simulink model "histogram_AXIS_TMI_2pix"  (R2015b)
settings: Solver=FixedStepDiscrete  SolverMode=SingleTasking  StartTime=0.0  StopTime=StartTime  FixedStep=1  RelTol=1e-3
values from neighbouring files (symbols this model uses):
  Nb_bin = 128    [Histogram_aldec_validation.m]    (also in Histogram_init.m = 1024; Histogram_init_20163.m; Histogram_init_validation.m)
  Ts = 1    [Histogram_aldec_validation.m]    (also in Histogram_init.m; Histogram_init_20163.m; Histogram_init_validation.m)
libraries: xbsIndex_r4 x128
settings Model: Creator=jboulet  LastModifiedBy=laboutilis
settings DataIOCC: SaveFormat=Array  SignalLoggingSaveFormat=ModelDataLogs
settings OptimizationCC: ExpressionDepthLimit=2147483647  InitFltsAndDblsToZero=on
settings DebuggingCC: AlgebraicLoopMsg=none  UnderspecifiedInitializationDetection=Classic  MergeDetectMultiDrivingBlocksExec=none  FcnCallInpInsideContextMsg=UseLocalSettings  UnconnectedInputMsg=none  UnconnectedOutputMsg=none  UnconnectedLineMsg=none  StateNameClashWarn=warning
settings HardwareCC: ProdBitPerPointer=32  ProdLargestAtomicFloat=None  ProdIntDivRoundTo=Undefined  ProdEndianess=Unspecified  ProdWordSize=32  ProdHWDeviceType=32-bit Generic
settings GRTTargetCC: GeneratePreprocessorConditionals=Disable all  CombineOutputUpdateFcns=off  GRTInterface=on
settings ConfigComp: CovModelRefEnable=Off

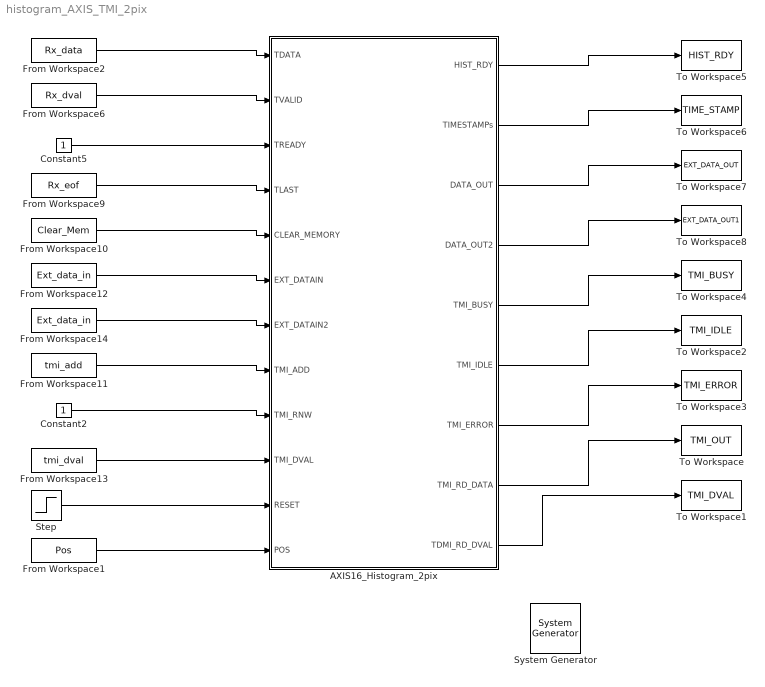
== system histogram_AXIS_TMI_2pix ==
  " System Generator" : xbsIndex_r4/ System Generator  Tag=genX  xilinxfamily=kintex7  part=xc7k160t  speed=-1  package=fbg676  synthesis_tool=Vivado  clock_wrapper=Clock Enables  directory=D:/Telops/FIR-00251-Proc/src/AEC/HDL/2pix_netlist_160  proj_type=Vivado  Synth_file=Vivado Synthesis Defaults  Impl_file=Vivado Implementation Defaults  testbench=off  simulink_period=1  sysclk_period=6.25  dcm_input_clock_period=10  incr_netlist=off  trim_vbits=Everywhere in SubSystem  dbl_ovrd=According to Block Masks  core_generation=According to Block Masks  run_coregen=off  deprecated_control=off  eval_field=0  block_type=sysgen
  AXIS16_Histogram_2pix : Subsystem
  Constant2 : Constant
  Constant5 : Constant
  From Workspace1 : FromWorkspace  VariableName=Pos  SampleTime=Ts  Interpolate=off  OutputAfterFinalValue=Holding final value
  From Workspace10 : FromWorkspace  VariableName=Clear_Mem  SampleTime=Ts  Interpolate=off  OutputAfterFinalValue=Setting to zero
  From Workspace11 : FromWorkspace  VariableName=tmi_add  SampleTime=Ts  Interpolate=off  OutputAfterFinalValue=Holding final value
  From Workspace12 : FromWorkspace  VariableName=Ext_data_in  SampleTime=Ts  Interpolate=off  OutputAfterFinalValue=Setting to zero
  From Workspace13 : FromWorkspace  VariableName=tmi_dval  SampleTime=Ts  Interpolate=off  OutputAfterFinalValue=Holding final value
  From Workspace14 : FromWorkspace  VariableName=Ext_data_in  SampleTime=Ts  Interpolate=off  OutputAfterFinalValue=Setting to zero
  From Workspace2 : FromWorkspace  VariableName=Rx_data  SampleTime=Ts  Interpolate=off  OutputAfterFinalValue=Setting to zero
  From Workspace6 : FromWorkspace  VariableName=Rx_dval  SampleTime=Ts  Interpolate=off  OutputAfterFinalValue=Setting to zero
  From Workspace9 : FromWorkspace  VariableName=Rx_eof  SampleTime=Ts  Interpolate=off  OutputAfterFinalValue=Setting to zero
  Step : Step  Time=5  Before=1  After=0  SampleTime=Ts
  To Workspace : ToWorkspace  VariableName=TMI_OUT  SampleTime=-1
  To Workspace1 : ToWorkspace  VariableName=TMI_DVAL  SampleTime=-1
  To Workspace2 : ToWorkspace  VariableName=TMI_IDLE  SampleTime=-1
  To Workspace3 : ToWorkspace  VariableName=TMI_ERROR  SampleTime=-1
  To Workspace4 : ToWorkspace  VariableName=TMI_BUSY  SampleTime=-1
  To Workspace5 : ToWorkspace  VariableName=HIST_RDY  SampleTime=-1
  To Workspace6 : ToWorkspace  VariableName=TIME_STAMP  SampleTime=-1
  To Workspace7 : ToWorkspace  VariableName=EXT_DATA_OUT  SampleTime=-1
  To Workspace8 : ToWorkspace  VariableName=EXT_DATA_OUT1  SampleTime=-1
  wires:
  From Workspace2/1 -> AXIS16_Histogram_2pix/1(TDATA)
  From Workspace6/1 -> AXIS16_Histogram_2pix/2(TVALID)
  Constant5/1 -> AXIS16_Histogram_2pix/3(TREADY)
  From Workspace9/1 -> AXIS16_Histogram_2pix/4(TLAST)
  From Workspace10/1 -> AXIS16_Histogram_2pix/5(CLEAR_MEMORY)
  From Workspace12/1 -> AXIS16_Histogram_2pix/6(EXT_DATAIN)
  From Workspace14/1 -> AXIS16_Histogram_2pix/7(EXT_DATAIN2)
  From Workspace11/1 -> AXIS16_Histogram_2pix/8(TMI_ADD)
  Constant2/1 -> AXIS16_Histogram_2pix/9(TMI_RNW)
  From Workspace13/1 -> AXIS16_Histogram_2pix/10(TMI_DVAL)
  AXIS16_Histogram_2pix/1(HIST_RDY) -> To Workspace5/1
  AXIS16_Histogram_2pix/2(TIMESTAMPs) -> To Workspace6/1
  AXIS16_Histogram_2pix/3(DATA_OUT) -> To Workspace7/1
  AXIS16_Histogram_2pix/4(DATA_OUT2) -> To Workspace8/1
  AXIS16_Histogram_2pix/5(TMI_BUSY) -> To Workspace4/1
  AXIS16_Histogram_2pix/6(TMI_IDLE) -> To Workspace2/1
  AXIS16_Histogram_2pix/7(TMI_ERROR) -> To Workspace3/1
  AXIS16_Histogram_2pix/8(TMI_RD_DATA) -> To Workspace/1
  AXIS16_Histogram_2pix/9(TDMI_RD_DVAL) -> To Workspace1/1
  Step/1 -> AXIS16_Histogram_2pix/11(RESET)
  From Workspace1/1 -> AXIS16_Histogram_2pix/12(POS)

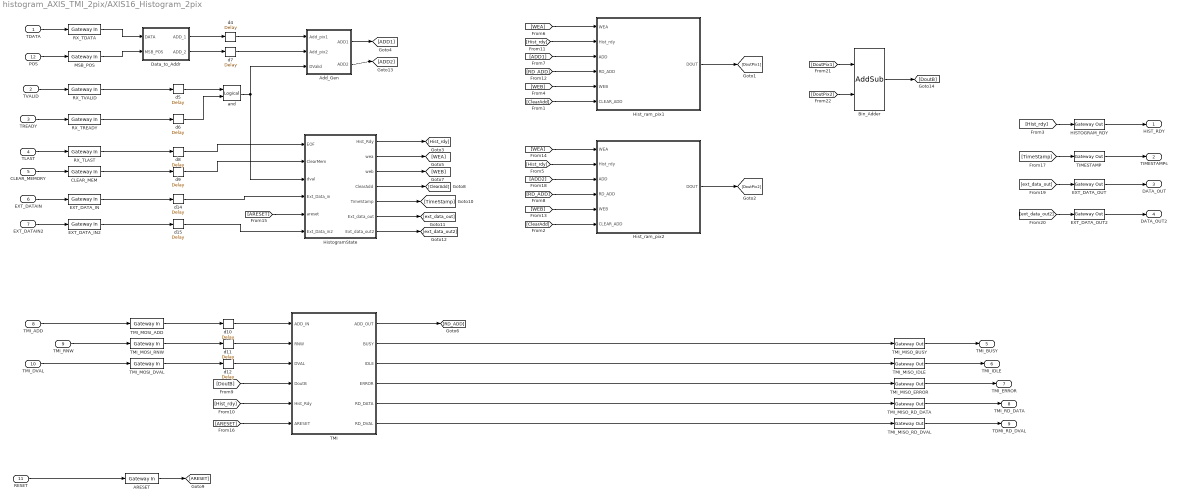
== system histogram_AXIS_TMI_2pix/AXIS16_Histogram_2pix ==
  TDATA : Inport
  TVALID : Inport  Port=2
  TREADY : Inport  Port=3
  TLAST : Inport  Port=4
  CLEAR_MEMORY : Inport  Port=5
  EXT_DATAIN : Inport  Port=6
  EXT_DATAIN2 : Inport  Port=7
  TMI_ADD : Inport  Port=8
  TMI_RNW : Inport  Port=9
  TMI_DVAL : Inport  Port=10
  RESET : Inport  Port=11
  POS : Inport  Port=12
  ARESET : xbsIndex_r4/Gateway In  gui_display_data_type=Boolean  arith_type=Boolean  n_bits=8  bin_pt=0  preci_type=Single  exp_width=8  frac_width=24  rows=1  columns=1  quantization="Round  (unbiased: +/- Inf)"  overflow=Wrap  period=1  UseAsADC=off  ADCChannel='1'  interface=None  automatic_assignment=on  address_offset=hex2dec('00')  intf_name=''  intf_description=''  default_value=0  timing_constraint=None  locs_specified=off  LOCs={}  io_standard={}  inherit_from_input=off  hdl_port=on  dbl_ovrd=off  block_type=gatewayin
      settings: xl_area=[0 0 0 0 1 0 0]  block_version=10.1.3
  Add_Gen : Subsystem
  Bin_Adder : xbsIndex_r4/AddSub  mode=Addition  use_carryin=off  use_carryout=off  en=off  latency=0  precision=User Defined  arith_type=Unsigned  n_bits=MaxHistValue_bit  bin_pt=0  quantization=Truncate  overflow=Wrap  use_behavioral_HDL=off  hw_selection=Fabric  pipelined=off  dbl_ovrd=off  block_type=addsub
  CLEAR_MEM : xbsIndex_r4/Gateway In  gui_display_data_type=Boolean  arith_type=Boolean  n_bits=8  bin_pt=0  preci_type=Single  exp_width=8  frac_width=24  rows=1  columns=1  quantization="Round  (unbiased: +/- Inf)"  overflow=Wrap  period=1  UseAsADC=off  ADCChannel='1'  interface=None  automatic_assignment=on  address_offset=hex2dec('00')  intf_name=''  intf_description=''  default_value=0  timing_constraint=None  locs_specified=off  LOCs={}  io_standard={}  inherit_from_input=off  hdl_port=on  dbl_ovrd=off  block_type=gatewayin
      settings: xl_area=[0 0 0 0 1 0 0]  block_version=10.1.3
  Data_to_Addr : Subsystem
  EXT_DATA_IN : xbsIndex_r4/Gateway In  gui_display_data_type=Fixed-point  arith_type=Unsigned  n_bits=32  bin_pt=0  preci_type=Single  exp_width=8  frac_width=24  rows=1  columns=1  quantization=Truncate  overflow=Wrap  period=1  UseAsADC=off  ADCChannel='1'  interface=None  automatic_assignment=on  address_offset=hex2dec('00')  intf_name=''  intf_description=''  default_value=0  timing_constraint=None  locs_specified=off  LOCs={}  io_standard={}  inherit_from_input=off  hdl_port=on  dbl_ovrd=off  block_type=gatewayin
      settings: xl_area=[0 0 0 0 1 0 0]  block_version=10.1.3
  EXT_DATA_IN2 : xbsIndex_r4/Gateway In  gui_display_data_type=Fixed-point  arith_type=Unsigned  n_bits=32  bin_pt=0  preci_type=Single  exp_width=8  frac_width=24  rows=1  columns=1  quantization=Truncate  overflow=Wrap  period=1  UseAsADC=off  ADCChannel='1'  interface=None  automatic_assignment=on  address_offset=hex2dec('00')  intf_name=''  intf_description=''  default_value=0  timing_constraint=None  locs_specified=off  LOCs={}  io_standard={}  inherit_from_input=off  hdl_port=on  dbl_ovrd=off  block_type=gatewayin
      settings: xl_area=[0 0 0 0 1 0 0]  block_version=10.1.3
  EXT_DATA_OUT : xbsIndex_r4/Gateway Out  inherit_from_input=off  hdl_port=on  rows=1  columns=1  UseAsDAC=off  DACChannel='1'  interface=None  automatic_assignment=on  address_offset=hex2dec('00')  intf_name=''  intf_description=''  timing_constraint=None  locs_specified=off  LOCs={}  io_standard={}  block_type=gatewayout
      settings: xl_area=[0 0 0 0 1 0 0]  block_version=10.1.3
  EXT_DATA_OUT2 : xbsIndex_r4/Gateway Out  inherit_from_input=off  hdl_port=on  rows=1  columns=1  UseAsDAC=off  DACChannel='1'  interface=None  automatic_assignment=on  address_offset=hex2dec('00')  intf_name=''  intf_description=''  timing_constraint=None  locs_specified=off  LOCs={}  io_standard={}  block_type=gatewayout
      settings: xl_area=[0 0 0 0 1 0 0]  block_version=10.1.3
  HISTOGRAM_RDY : xbsIndex_r4/Gateway Out  inherit_from_input=off  hdl_port=on  rows=1  columns=1  UseAsDAC=off  DACChannel='1'  interface=None  automatic_assignment=on  address_offset=hex2dec('00')  intf_name=''  intf_description=''  timing_constraint=None  locs_specified=off  LOCs={}  io_standard={}  block_type=gatewayout
      settings: xl_area=[0 0 0 0 1 0 0]  block_version=10.1.3
  Hist_ram_pix1 : Subsystem
  Hist_ram_pix2 : Subsystem
  HistogramState : Subsystem
  MSB_POS : xbsIndex_r4/Gateway In  gui_display_data_type=Fixed-point  arith_type=Unsigned  n_bits=2  bin_pt=0  preci_type=Single  exp_width=8  frac_width=24  rows=1  columns=1  quantization=Truncate  overflow=Wrap  period=Ts  UseAsADC=off  ADCChannel='1'  interface=None  automatic_assignment=on  address_offset=hex2dec('00')  intf_name=''  intf_description=''  default_value=0  timing_constraint=None  locs_specified=off  LOCs={}  io_standard={}  inherit_from_input=off  hdl_port=on  dbl_ovrd=off  block_type=gatewayin
      settings: xl_area=[0 0 0 0 1 0 0]  block_version=10.1.3
  RX_TDATA : xbsIndex_r4/Gateway In  gui_display_data_type=Fixed-point  arith_type=Unsigned  n_bits=32  bin_pt=0  preci_type=Single  exp_width=8  frac_width=24  rows=1  columns=1  quantization="Round  (unbiased: +/- Inf)"  overflow=Wrap  period=Ts  UseAsADC=off  ADCChannel='1'  interface=None  automatic_assignment=on  address_offset=hex2dec('00')  intf_name=''  intf_description=''  default_value=0  timing_constraint=None  locs_specified=off  LOCs={}  io_standard={}  inherit_from_input=off  hdl_port=on  dbl_ovrd=off  block_type=gatewayin
      settings: xl_area=[0 0 0 0 10 0 0]  block_version=10.1.3
  RX_TLAST : xbsIndex_r4/Gateway In  gui_display_data_type=Boolean  arith_type=Boolean  n_bits=8  bin_pt=0  preci_type=Single  exp_width=8  frac_width=24  rows=1  columns=1  quantization="Round  (unbiased: +/- Inf)"  overflow=Wrap  period=1  UseAsADC=off  ADCChannel='1'  interface=None  automatic_assignment=on  address_offset=hex2dec('00')  intf_name=''  intf_description=''  default_value=0  timing_constraint=None  locs_specified=off  LOCs={}  io_standard={}  inherit_from_input=off  hdl_port=on  dbl_ovrd=off  block_type=gatewayin
      settings: xl_area=[0 0 0 0 1 0 0]  block_version=10.1.3
  RX_TREADY : xbsIndex_r4/Gateway In  gui_display_data_type=Boolean  arith_type=Boolean  n_bits=8  bin_pt=0  preci_type=Single  exp_width=8  frac_width=24  rows=1  columns=1  quantization="Round  (unbiased: +/- Inf)"  overflow=Wrap  period=1  UseAsADC=off  ADCChannel='1'  interface=None  automatic_assignment=on  address_offset=hex2dec('00')  intf_name=''  intf_description=''  default_value=0  timing_constraint=None  locs_specified=off  LOCs={}  io_standard={}  inherit_from_input=off  hdl_port=on  dbl_ovrd=off  block_type=gatewayin
      settings: xl_area=[0 0 0 0 1 0 0]  block_version=10.1.3
  RX_TVALID : xbsIndex_r4/Gateway In  gui_display_data_type=Boolean  arith_type=Boolean  n_bits=8  bin_pt=0  preci_type=Single  exp_width=8  frac_width=24  rows=1  columns=1  quantization="Round  (unbiased: +/- Inf)"  overflow=Wrap  period=1  UseAsADC=off  ADCChannel='1'  interface=None  automatic_assignment=on  address_offset=hex2dec('00')  intf_name=''  intf_description=''  default_value=0  timing_constraint=None  locs_specified=off  LOCs={}  io_standard={}  inherit_from_input=off  hdl_port=on  dbl_ovrd=off  block_type=gatewayin
      settings: xl_area=[0 0 0 0 1 0 0]  block_version=10.1.3
  TIMESTAMP : xbsIndex_r4/Gateway Out  inherit_from_input=off  hdl_port=on  rows=1  columns=1  UseAsDAC=off  DACChannel='1'  interface=None  automatic_assignment=on  address_offset=hex2dec('00')  intf_name=''  intf_description=''  timing_constraint=None  locs_specified=off  LOCs={}  io_standard={}  block_type=gatewayout
      settings: xl_area=[0 0 0 0 1 0 0]  block_version=10.1.3
  TMI : Subsystem
  TMI_MISO_BUSY : xbsIndex_r4/Gateway Out  inherit_from_input=off  hdl_port=on  rows=1  columns=1  UseAsDAC=off  DACChannel='1'  interface=None  automatic_assignment=on  address_offset=hex2dec('00')  intf_name=''  intf_description=''  timing_constraint=None  locs_specified=off  LOCs={}  io_standard={}  block_type=gatewayout
      settings: xl_area=[0 0 0 0 1 0 0]  block_version=10.1.3
  TMI_MISO_ERROR : xbsIndex_r4/Gateway Out  inherit_from_input=off  hdl_port=on  rows=1  columns=1  UseAsDAC=off  DACChannel='1'  interface=None  automatic_assignment=on  address_offset=hex2dec('00')  intf_name=''  intf_description=''  timing_constraint=None  locs_specified=off  LOCs={}  io_standard={}  block_type=gatewayout
      settings: xl_area=[0 0 0 0 1 0 0]  block_version=10.1.3
  TMI_MISO_IDLE : xbsIndex_r4/Gateway Out  inherit_from_input=off  hdl_port=on  rows=1  columns=1  UseAsDAC=off  DACChannel='1'  interface=None  automatic_assignment=on  address_offset=hex2dec('00')  intf_name=''  intf_description=''  timing_constraint=None  locs_specified=off  LOCs={}  io_standard={}  block_type=gatewayout
      settings: xl_area=[0 0 0 0 1 0 0]  block_version=10.1.3
  TMI_MISO_RD_DATA : xbsIndex_r4/Gateway Out  inherit_from_input=off  hdl_port=on  rows=1  columns=1  UseAsDAC=off  DACChannel='1'  interface=None  automatic_assignment=on  address_offset=hex2dec('00')  intf_name=''  intf_description=''  timing_constraint=None  locs_specified=off  LOCs={}  io_standard={}  block_type=gatewayout
      settings: xl_area=[0 0 0 0 21 0 0]  block_version=10.1.3
  TMI_MISO_RD_DVAL : xbsIndex_r4/Gateway Out  inherit_from_input=off  hdl_port=on  rows=1  columns=1  UseAsDAC=off  DACChannel='1'  interface=None  automatic_assignment=on  address_offset=hex2dec('00')  intf_name=''  intf_description=''  timing_constraint=None  locs_specified=off  LOCs={}  io_standard={}  block_type=gatewayout
      settings: xl_area=[0 0 0 0 1 0 0]  block_version=10.1.3
  TMI_MOSI_ADD : xbsIndex_r4/Gateway In  gui_display_data_type=Fixed-point  arith_type=Unsigned  n_bits=log2(Nb_bin)  bin_pt=0  preci_type=Single  exp_width=8  frac_width=24  rows=1  columns=1  quantization=Truncate  overflow=Wrap  period=Ts  UseAsADC=off  ADCChannel='1'  interface=None  automatic_assignment=on  address_offset=hex2dec('00')  intf_name=''  intf_description=''  default_value=0  timing_constraint=None  locs_specified=off  LOCs={}  io_standard={}  inherit_from_input=off  hdl_port=on  dbl_ovrd=off  block_type=gatewayin
      settings: xl_area=[0 0 0 0 4 0 0]  block_version=10.1.3
  TMI_MOSI_DVAL : xbsIndex_r4/Gateway In  gui_display_data_type=Boolean  arith_type=Boolean  n_bits=8  bin_pt=0  preci_type=Single  exp_width=8  frac_width=24  rows=1  columns=1  quantization="Round  (unbiased: +/- Inf)"  overflow=Wrap  period=1  UseAsADC=off  ADCChannel='1'  interface=None  automatic_assignment=on  address_offset=hex2dec('00')  intf_name=''  intf_description=''  default_value=0  timing_constraint=None  locs_specified=off  LOCs={}  io_standard={}  inherit_from_input=off  hdl_port=on  dbl_ovrd=off  block_type=gatewayin
      settings: xl_area=[0 0 0 0 1 0 0]  block_version=10.1.3
  TMI_MOSI_RNW : xbsIndex_r4/Gateway In  gui_display_data_type=Boolean  arith_type=Boolean  n_bits=8  bin_pt=0  preci_type=Single  exp_width=8  frac_width=24  rows=1  columns=1  quantization="Round  (unbiased: +/- Inf)"  overflow=Wrap  period=1  UseAsADC=off  ADCChannel='1'  interface=None  automatic_assignment=on  address_offset=hex2dec('00')  intf_name=''  intf_description=''  default_value=0  timing_constraint=None  locs_specified=off  LOCs={}  io_standard={}  inherit_from_input=off  hdl_port=on  dbl_ovrd=off  block_type=gatewayin
      settings: xl_area=[0 0 0 0 1 0 0]  block_version=10.1.3
  and : xbsIndex_r4/Logical  logical_function=AND  inputs=2  en=off  latency=0  precision=Full  arith_type=Unsigned  n_bits=16  bin_pt=0  align_bp=on  dbl_ovrd=off  block_type=logical
      settings: xl_area=[1 0 0 1 0 0 0]
  d{4..12,14..15} (11 alike) : xbsIndex_r4/Delay  rst=off  infoeditControl=Selection of Reset will increase slice count due to use of real FFs and instead of SRLs  en=off  latency=1  reg_retiming=off  dbl_ovrd=off  block_type=delay
      d10 settings: xl_area=[2 4 0 0 0 0 0]
      d11 settings: xl_area=[1 1 0 0 0 0 0]
      d12 settings: xl_area=[1 1 0 0 0 0 0]
      d14 settings: xl_area=[1 1 0 0 0 0 0]
      d15 settings: xl_area=[1 1 0 0 0 0 0]
      d4 settings: xl_area=[5 10 0 0 0 0 0]
      d5 settings: xl_area=[1 1 0 0 0 0 0]
      d6 settings: xl_area=[1 1 0 0 0 0 0]
      d7 settings: xl_area=[5 10 0 0 0 0 0]
      d8 settings: xl_area=[1 1 0 0 0 0 0]
      d9 settings: xl_area=[1 1 0 0 0 0 0]
  HIST_RDY : Outport
  TIMESTAMPs : Outport  Port=2
  DATA_OUT : Outport  Port=3
  DATA_OUT2 : Outport  Port=4
  TMI_BUSY : Outport  Port=5
  TMI_IDLE : Outport  Port=6
  TMI_ERROR : Outport  Port=7
  TMI_RD_DATA : Outport  Port=8
  TDMI_RD_DVAL : Outport  Port=9
  wires:
  [ARESET] -> HistogramState/5(areset)
  [ARESET] -> TMI/6(ARESET)
  ARESET/1 -> [ARESET]
  TMI_MOSI_ADD/1 -> d10/1
  TMI_MOSI_DVAL/1 -> d12/1
  d10/1 -> TMI/1(ADD_IN)
  [DoutB] -> TMI/4(DoutB)
  [Hist_rdy] -> TMI/5(Hist_Rdy)
  TMI/1(ADD_OUT) -> [RD_ADD]
  TMI_MOSI_RNW/1 -> d11/1
  TMI/2(BUSY) -> TMI_MISO_BUSY/1
  TMI/4(ERROR) -> TMI_MISO_ERROR/1
  TMI/5(RD_DATA) -> TMI_MISO_RD_DATA/1
  HistogramState/4(ClearAdd) -> [ClearAdd]
  TMI/6(RD_DVAL) -> TMI_MISO_RD_DVAL/1
  TMI_ADD/1 -> TMI_MOSI_ADD/1
  TMI_RNW/1 -> TMI_MOSI_RNW/1
  TMI_DVAL/1 -> TMI_MOSI_DVAL/1
  HistogramState/3(web) -> [WEB]
  TMI/3(IDLE) -> TMI_MISO_IDLE/1
  d12/1 -> TMI/3(DVAL)
  d11/1 -> TMI/2(RNW)
  HistogramState/5(TimeStamp) -> [TimeStamp]
  [TimeStamp] -> TIMESTAMP/1
  TMI_MISO_RD_DVAL/1 -> TDMI_RD_DVAL/1
  TMI_MISO_RD_DATA/1 -> TMI_RD_DATA/1
  [ext_data_out2] -> EXT_DATA_OUT2/1
  HistogramState/7(Ext_data_out2) -> [ext_data_out2]
  d15/1 -> HistogramState/6(Ext_Data_in2)
  EXT_DATA_IN2/1 -> d15/1
  [ext_data_out] -> EXT_DATA_OUT/1
  HistogramState/6(Ext_data_out) -> [ext_data_out]
  d14/1 -> HistogramState/4(Ext_Data_in)
  EXT_DATA_IN/1 -> d14/1
  HistogramState/2(wea) -> [WEA]
  d8/1 -> HistogramState/1(EOF)
  RESET/1 -> ARESET/1
  [Hist_rdy] -> HISTOGRAM_RDY/1
  d9/1 -> HistogramState/2(ClearMem)
  d5/1 -> and/1
  HistogramState/1(Hist_Rdy) -> [Hist_rdy]
  TDATA/1 -> RX_TDATA/1
  and/1 -> Add_Gen/3(DValid), HistogramState/3(dval)
  RX_TLAST/1 -> d8/1
  CLEAR_MEM/1 -> d9/1
  TVALID/1 -> RX_TVALID/1
  RX_TREADY/1 -> d6/1
  CLEAR_MEMORY/1 -> CLEAR_MEM/1
  TREADY/1 -> RX_TREADY/1
  TLAST/1 -> RX_TLAST/1
  RX_TVALID/1 -> d5/1
  d6/1 -> and/2
  TMI_MISO_BUSY/1 -> TMI_BUSY/1
  EXT_DATA_OUT/1 -> DATA_OUT/1
  EXT_DATAIN/1 -> EXT_DATA_IN/1
  TMI_MISO_ERROR/1 -> TMI_ERROR/1
  TMI_MISO_IDLE/1 -> TMI_IDLE/1
  EXT_DATA_OUT2/1 -> DATA_OUT2/1
  TIMESTAMP/1 -> TIMESTAMPs/1
  HISTOGRAM_RDY/1 -> HIST_RDY/1
  EXT_DATAIN2/1 -> EXT_DATA_IN2/1
  POS/1 -> MSB_POS/1
  Data_to_Addr/1(ADD_1) -> d4/1
  RX_TDATA/1 -> Data_to_Addr/1(DATA)
  MSB_POS/1 -> Data_to_Addr/2(MSB_POS)
  d4/1 -> Add_Gen/1(Add_pix1)
  Add_Gen/1(ADD1) -> [ADD1]
  Data_to_Addr/2(ADD_2) -> d7/1
  d7/1 -> Add_Gen/2(Add_pix2)
  Add_Gen/2(ADD2) -> [ADD2]
  [WEA] -> Hist_ram_pix1/1(WEA)
  [Hist_rdy] -> Hist_ram_pix1/2(Hist_rdy)
  [ADD1] -> Hist_ram_pix1/3(ADD)
  [RD_ADD] -> Hist_ram_pix1/4(RD_ADD)
  [WEB] -> Hist_ram_pix1/5(WEB)
  Hist_ram_pix1/1(DOUT) -> [DoutPix1]
  [ClearAdd] -> Hist_ram_pix1/6(CLEAR_ADD)
  [ClearAdd] -> Hist_ram_pix2/6(CLEAR_ADD)
  [WEB] -> Hist_ram_pix2/5(WEB)
  [RD_ADD] -> Hist_ram_pix2/4(RD_ADD)
  [WEA] -> Hist_ram_pix2/1(WEA)
  [Hist_rdy] -> Hist_ram_pix2/2(Hist_rdy)
  [ADD2] -> Hist_ram_pix2/3(ADD)
  Hist_ram_pix2/1(DOUT) -> [DoutPix2]
  [DoutPix1] -> Bin_Adder/1
  [DoutPix2] -> Bin_Adder/2
  Bin_Adder/1 -> [DoutB]

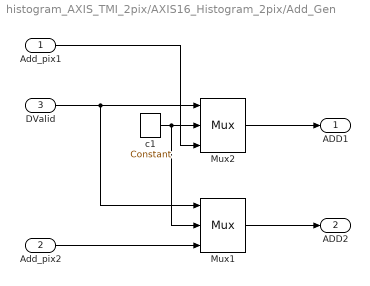
== system histogram_AXIS_TMI_2pix/AXIS16_Histogram_2pix/Add_Gen ==
  Add_pix1 : Inport
  Add_pix2 : Inport  Port=2
  DValid : Inport  Port=3
  Mux1 : xbsIndex_r4/Mux  inputs=2  en=off  latency=0  precision=Full  arith_type=Unsigned  n_bits=16  bin_pt=14  quantization=Truncate  overflow=Wrap  dbl_ovrd=off  block_type=mux
      settings: xl_area=[2 0 0 4 0 0 0]
  Mux2 : xbsIndex_r4/Mux  inputs=2  en=off  latency=0  precision=Full  arith_type=Unsigned  n_bits=16  bin_pt=14  quantization=Truncate  overflow=Wrap  dbl_ovrd=off  block_type=mux
      settings: xl_area=[2 0 0 4 0 0 0]
  c1 : xbsIndex_r4/Constant  const=0  gui_display_data_type=Fixed-point  arith_type=Unsigned  n_bits=log2(Nb_bin)  bin_pt=0  preci_type=Single  exp_width=8  frac_width=24  explicit_period=off  period=1  equ=P=C  opselect=C  inp2=PCIN>>17  opr=+  inp1=P  carry=CIN  dbl_ovrd=off  block_type=constant
  ADD1 : Outport
  ADD2 : Outport  Port=2
  wires:
  DValid/1 -> Mux1/1, Mux2/1
  Mux2/1 -> ADD1/1
  c1/1 -> Mux1/2, Mux2/2
  Add_pix1/1 -> Mux2/3
  Add_pix2/1 -> Mux1/3
  Mux1/1 -> ADD2/1

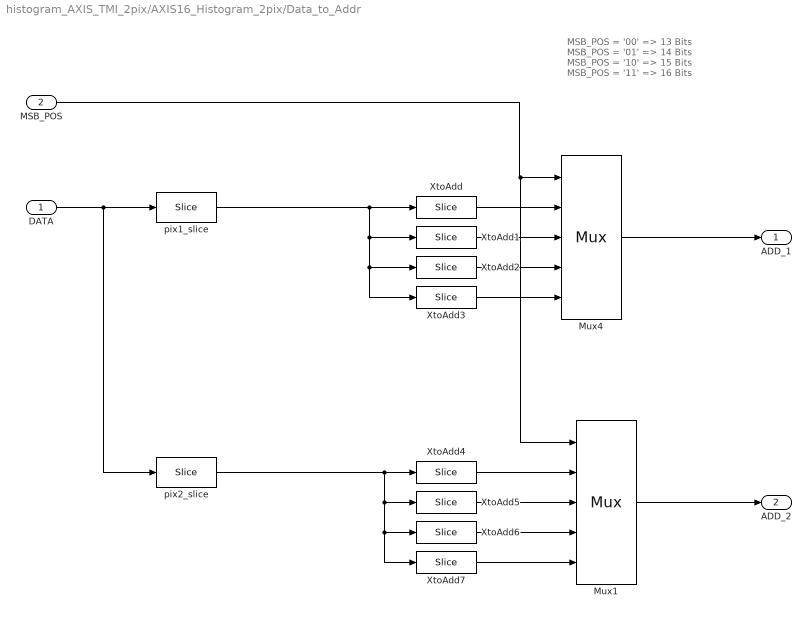
== system histogram_AXIS_TMI_2pix/AXIS16_Histogram_2pix/Data_to_Addr ==
  note: MSB_POS = '00' => 13 Bits
      | MSB_POS = '01' => 14 Bits
      | MSB_POS = '10' => 15 Bits
      | MSB_POS = '11' => 16 Bits
  DATA : Inport
  MSB_POS : Inport  Port=2
  Mux1 : xbsIndex_r4/Mux  inputs=4  en=off  latency=0  precision=Full  arith_type=Unsigned  n_bits=16  bin_pt=14  quantization=Truncate  overflow=Wrap  dbl_ovrd=off  block_type=mux
      settings: xl_area=[2 0 0 4 0 0 0]
  Mux4 : xbsIndex_r4/Mux  inputs=4  en=off  latency=0  precision=Full  arith_type=Unsigned  n_bits=16  bin_pt=14  quantization=Truncate  overflow=Wrap  dbl_ovrd=off  block_type=mux
      settings: xl_area=[2 0 0 4 0 0 0]
  XtoAdd : xbsIndex_r4/Slice  nbits=log2(Nb_bin)  boolean_output=off  mode=Upper Bit Location + Width  bit1=-3  base1=MSB of Input  bit0=0  base0=LSB of Input  dbl_ovrd=off  block_type=slice
      settings: block_version=10.1.3
  XtoAdd1 : xbsIndex_r4/Slice  nbits=log2(Nb_bin)  boolean_output=off  mode=Upper Bit Location + Width  bit1=-2  base1=MSB of Input  bit0=0  base0=LSB of Input  dbl_ovrd=off  block_type=slice
      settings: block_version=10.1.3
  XtoAdd2 : xbsIndex_r4/Slice  nbits=log2(Nb_bin)  boolean_output=off  mode=Upper Bit Location + Width  bit1=-1  base1=MSB of Input  bit0=0  base0=LSB of Input  dbl_ovrd=off  block_type=slice
      settings: block_version=10.1.3
  XtoAdd3 : xbsIndex_r4/Slice  nbits=log2(Nb_bin)  boolean_output=off  mode=Upper Bit Location + Width  bit1=0  base1=MSB of Input  bit0=0  base0=LSB of Input  dbl_ovrd=off  block_type=slice
      settings: block_version=10.1.3
  XtoAdd4 : xbsIndex_r4/Slice  nbits=log2(Nb_bin)  boolean_output=off  mode=Upper Bit Location + Width  bit1=-3  base1=MSB of Input  bit0=0  base0=LSB of Input  dbl_ovrd=off  block_type=slice
      settings: block_version=10.1.3
  XtoAdd5 : xbsIndex_r4/Slice  nbits=log2(Nb_bin)  boolean_output=off  mode=Upper Bit Location + Width  bit1=-2  base1=MSB of Input  bit0=0  base0=LSB of Input  dbl_ovrd=off  block_type=slice
      settings: block_version=10.1.3
  XtoAdd6 : xbsIndex_r4/Slice  nbits=log2(Nb_bin)  boolean_output=off  mode=Upper Bit Location + Width  bit1=-1  base1=MSB of Input  bit0=0  base0=LSB of Input  dbl_ovrd=off  block_type=slice
      settings: block_version=10.1.3
  XtoAdd7 : xbsIndex_r4/Slice  nbits=log2(Nb_bin)  boolean_output=off  mode=Upper Bit Location + Width  bit1=0  base1=MSB of Input  bit0=0  base0=LSB of Input  dbl_ovrd=off  block_type=slice
      settings: block_version=10.1.3
  pix1_slice : xbsIndex_r4/Slice  nbits=16  boolean_output=off  mode=Lower Bit Location + Width  bit1=0  base1=MSB of Input  bit0=0  base0=LSB of Input  dbl_ovrd=off  block_type=slice
  pix2_slice : xbsIndex_r4/Slice  nbits=16  boolean_output=off  mode=Lower Bit Location + Width  bit1=0  base1=MSB of Input  bit0=16  base0=LSB of Input  dbl_ovrd=off  block_type=slice
  ADD_1 : Outport
  ADD_2 : Outport  Port=2
  wires:
  Mux4/1 -> ADD_1/1
  MSB_POS/1 -> Mux1/1, Mux4/1
  XtoAdd/1 -> Mux4/2
  XtoAdd1/1 -> Mux4/3
  DATA/1 -> pix2_slice/1, pix1_slice/1
  XtoAdd2/1 -> Mux4/4
  XtoAdd3/1 -> Mux4/5
  pix1_slice/1 -> XtoAdd2/1, XtoAdd3/1, XtoAdd1/1, XtoAdd/1
  XtoAdd4/1 -> Mux1/2
  XtoAdd5/1 -> Mux1/3
  XtoAdd6/1 -> Mux1/4
  XtoAdd7/1 -> Mux1/5
  pix2_slice/1 -> XtoAdd7/1, XtoAdd6/1, XtoAdd5/1, XtoAdd4/1
  Mux1/1 -> ADD_2/1

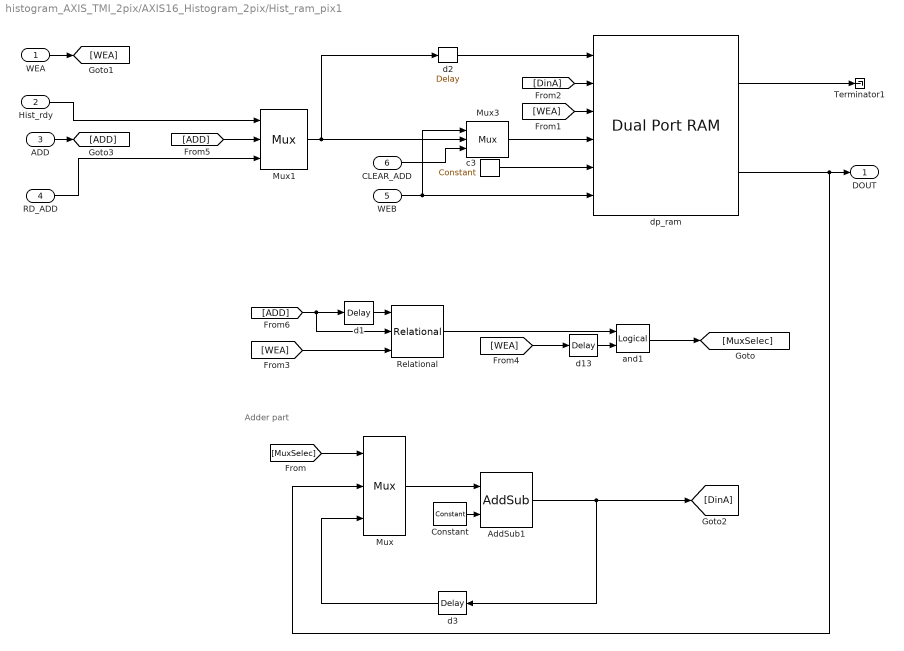
== system histogram_AXIS_TMI_2pix/AXIS16_Histogram_2pix/Hist_ram_pix1 ==
  note: Adder part
  WEA : Inport
  Hist_rdy : Inport  Port=2
  ADD : Inport  Port=3
  RD_ADD : Inport  Port=4
  WEB : Inport  Port=5
  CLEAR_ADD : Inport  Port=6
  AddSub1 : xbsIndex_r4/AddSub  mode=Addition  use_carryin=off  use_carryout=off  en=off  latency=0  precision=User Defined  arith_type=Unsigned  n_bits=MaxHistValue_bit  bin_pt=0  quantization=Truncate  overflow=Wrap  use_behavioral_HDL=off  hw_selection=Fabric  pipelined=off  dbl_ovrd=off  block_type=addsub
  Constant : xbsIndex_r4/Constant  const=1  gui_display_data_type=Fixed-point  arith_type=Unsigned  n_bits=1  bin_pt=0  preci_type=Single  exp_width=8  frac_width=24  explicit_period=off  period=1  equ=P=C  opselect=C  inp2=PCIN>>17  opr=+  inp1=P  carry=CIN  dbl_ovrd=off  block_type=constant
  Mux : xbsIndex_r4/Mux  inputs=2  en=off  latency=0  precision=Full  arith_type=Unsigned  n_bits=16  bin_pt=14  quantization=Truncate  overflow=Wrap  dbl_ovrd=off  block_type=mux
      settings: xl_area=[11 0 0 21 0 0 0]
  Mux1 : xbsIndex_r4/Mux  inputs=2  en=off  latency=0  precision=Full  arith_type=Unsigned  n_bits=16  bin_pt=14  quantization=Truncate  overflow=Wrap  dbl_ovrd=off  block_type=mux
      settings: xl_area=[2 0 0 4 0 0 0]
  Mux3 : xbsIndex_r4/Mux  inputs=2  en=off  latency=0  precision=Full  arith_type=Unsigned  n_bits=16  bin_pt=14  quantization=Truncate  overflow=Wrap  dbl_ovrd=off  block_type=mux
      settings: xl_area=[2 0 0 4 0 0 0]
  Relational : xbsIndex_r4/Relational  mode=a=b  op_type=Bool  en=on  latency=1  dbl_ovrd=off  block_type=relational
      settings: xl_area=[1 1 0 2 0 0 0]  block_version=10.1.3
  Terminator1 : Terminator
  and1 : xbsIndex_r4/Logical  logical_function=AND  inputs=2  en=off  latency=0  precision=Full  arith_type=Unsigned  n_bits=16  bin_pt=0  align_bp=on  dbl_ovrd=off  block_type=logical
      settings: xl_area=[1 0 0 1 0 0 0]
  c3 : xbsIndex_r4/Constant  const=0  gui_display_data_type=Fixed-point  arith_type=Unsigned  n_bits=MaxHistValue_bit  bin_pt=0  preci_type=Single  exp_width=8  frac_width=24  explicit_period=off  period=1  equ=P=C  opselect=C  inp2=PCIN>>17  opr=+  inp1=P  carry=CIN  dbl_ovrd=off  block_type=constant
  d{1..3,13} (4 alike) : xbsIndex_r4/Delay  rst=off  infoeditControl=Selection of Reset will increase slice count due to use of real FFs and instead of SRLs  en=off  latency=1  reg_retiming=off  dbl_ovrd=off  block_type=delay
      d1 settings: xl_area=[2 4 0 0 0 0 0]
      d13 settings: xl_area=[2 4 0 0 0 0 0]
      d2 settings: xl_area=[2 4 0 0 0 0 0]
      d3 settings: xl_area=[11 21 0 0 0 0 0]
  dp_ram : xbsIndex_r4/Dual Port RAM  depth=Nb_bin  initVector=0  distributed_mem=Block RAM  init_a=0  init_b=0  rst_a=off  rst_b=off  en_a=off  en_b=off  latency=1  write_mode_A=Read Before Write  write_mode_B=Read Before Write  optimize=Area  dbl_ovrd=off  block_type=dpram
  DOUT : Outport
  wires:
  AddSub1/1 -> [DinA], d3/1
  WEB/1 -> Mux3/1, dp_ram/6
  Mux3/1 -> dp_ram/4
  Mux1/1 -> d2/1, Mux3/2
  Hist_rdy/1 -> Mux1/1
  RD_ADD/1 -> Mux1/3
  and1/1 -> [MuxSelec]
  Relational/1 -> and1/1
  [WEA] -> d13/1
  d13/1 -> and1/2
  [ADD] -> d1/1, Relational/2
  [MuxSelec] -> Mux/1
  Mux/1 -> AddSub1/1
  Constant/1 -> AddSub1/2
  d3/1 -> Mux/3
  [WEA] -> Relational/3
  d1/1 -> Relational/1
  dp_ram/1 -> Terminator1/1
  dp_ram/2 -> Mux/2, DOUT/1
  c3/1 -> dp_ram/5
  d2/1 -> dp_ram/1
  [DinA] -> dp_ram/2
  WEA/1 -> [WEA]
  [WEA] -> dp_ram/3
  ADD/1 -> [ADD]
  [ADD] -> Mux1/2
  CLEAR_ADD/1 -> Mux3/3

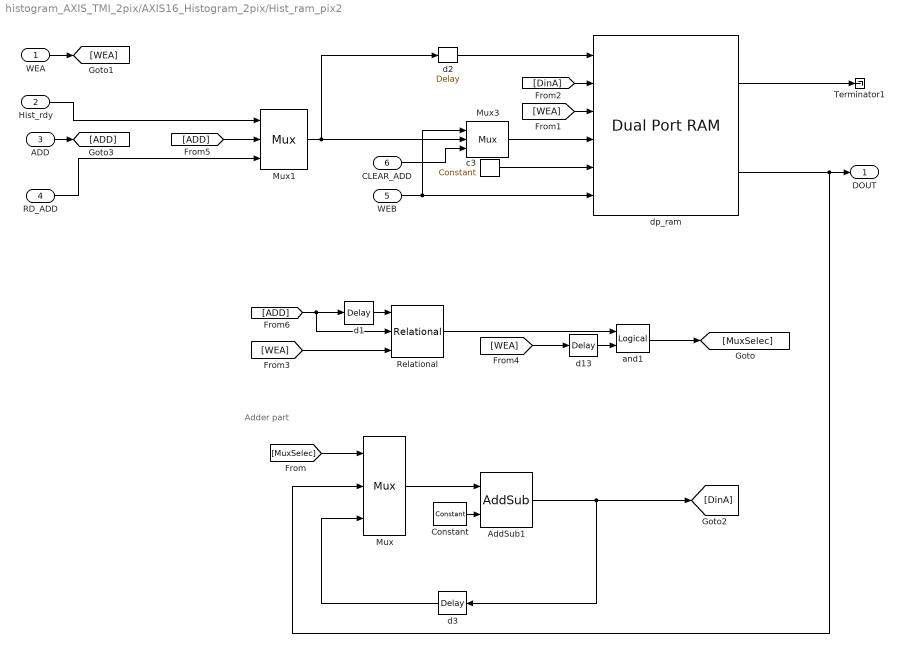
== system histogram_AXIS_TMI_2pix/AXIS16_Histogram_2pix/Hist_ram_pix2 ==
  note: Adder part
  WEA : Inport
  Hist_rdy : Inport  Port=2
  ADD : Inport  Port=3
  RD_ADD : Inport  Port=4
  WEB : Inport  Port=5
  CLEAR_ADD : Inport  Port=6
  AddSub1 : xbsIndex_r4/AddSub  mode=Addition  use_carryin=off  use_carryout=off  en=off  latency=0  precision=User Defined  arith_type=Unsigned  n_bits=MaxHistValue_bit  bin_pt=0  quantization=Truncate  overflow=Wrap  use_behavioral_HDL=off  hw_selection=Fabric  pipelined=off  dbl_ovrd=off  block_type=addsub
  Constant : xbsIndex_r4/Constant  const=1  gui_display_data_type=Fixed-point  arith_type=Unsigned  n_bits=1  bin_pt=0  preci_type=Single  exp_width=8  frac_width=24  explicit_period=off  period=1  equ=P=C  opselect=C  inp2=PCIN>>17  opr=+  inp1=P  carry=CIN  dbl_ovrd=off  block_type=constant
  Mux : xbsIndex_r4/Mux  inputs=2  en=off  latency=0  precision=Full  arith_type=Unsigned  n_bits=16  bin_pt=14  quantization=Truncate  overflow=Wrap  dbl_ovrd=off  block_type=mux
      settings: xl_area=[11 0 0 21 0 0 0]
  Mux1 : xbsIndex_r4/Mux  inputs=2  en=off  latency=0  precision=Full  arith_type=Unsigned  n_bits=16  bin_pt=14  quantization=Truncate  overflow=Wrap  dbl_ovrd=off  block_type=mux
      settings: xl_area=[2 0 0 4 0 0 0]
  Mux3 : xbsIndex_r4/Mux  inputs=2  en=off  latency=0  precision=Full  arith_type=Unsigned  n_bits=16  bin_pt=14  quantization=Truncate  overflow=Wrap  dbl_ovrd=off  block_type=mux
      settings: xl_area=[2 0 0 4 0 0 0]
  Relational : xbsIndex_r4/Relational  mode=a=b  op_type=Bool  en=on  latency=1  dbl_ovrd=off  block_type=relational
      settings: xl_area=[1 1 0 2 0 0 0]  block_version=10.1.3
  Terminator1 : Terminator
  and1 : xbsIndex_r4/Logical  logical_function=AND  inputs=2  en=off  latency=0  precision=Full  arith_type=Unsigned  n_bits=16  bin_pt=0  align_bp=on  dbl_ovrd=off  block_type=logical
      settings: xl_area=[1 0 0 1 0 0 0]
  c3 : xbsIndex_r4/Constant  const=0  gui_display_data_type=Fixed-point  arith_type=Unsigned  n_bits=MaxHistValue_bit  bin_pt=0  preci_type=Single  exp_width=8  frac_width=24  explicit_period=off  period=1  equ=P=C  opselect=C  inp2=PCIN>>17  opr=+  inp1=P  carry=CIN  dbl_ovrd=off  block_type=constant
  d{1..3,13} (4 alike) : xbsIndex_r4/Delay  rst=off  infoeditControl=Selection of Reset will increase slice count due to use of real FFs and instead of SRLs  en=off  latency=1  reg_retiming=off  dbl_ovrd=off  block_type=delay
      d1 settings: xl_area=[2 4 0 0 0 0 0]
      d13 settings: xl_area=[2 4 0 0 0 0 0]
      d2 settings: xl_area=[2 4 0 0 0 0 0]
      d3 settings: xl_area=[11 21 0 0 0 0 0]
  dp_ram : xbsIndex_r4/Dual Port RAM  depth=Nb_bin  initVector=0  distributed_mem=Block RAM  init_a=0  init_b=0  rst_a=off  rst_b=off  en_a=off  en_b=off  latency=1  write_mode_A=Read Before Write  write_mode_B=Read Before Write  optimize=Area  dbl_ovrd=off  block_type=dpram
  DOUT : Outport
  wires:
  AddSub1/1 -> [DinA], d3/1
  WEB/1 -> Mux3/1, dp_ram/6
  Mux3/1 -> dp_ram/4
  Mux1/1 -> d2/1, Mux3/2
  Hist_rdy/1 -> Mux1/1
  RD_ADD/1 -> Mux1/3
  and1/1 -> [MuxSelec]
  Relational/1 -> and1/1
  [WEA] -> d13/1
  d13/1 -> and1/2
  [ADD] -> d1/1, Relational/2
  [MuxSelec] -> Mux/1
  Mux/1 -> AddSub1/1
  Constant/1 -> AddSub1/2
  d3/1 -> Mux/3
  [WEA] -> Relational/3
  d1/1 -> Relational/1
  dp_ram/1 -> Terminator1/1
  dp_ram/2 -> Mux/2, DOUT/1
  c3/1 -> dp_ram/5
  d2/1 -> dp_ram/1
  [DinA] -> dp_ram/2
  WEA/1 -> [WEA]
  [WEA] -> dp_ram/3
  ADD/1 -> [ADD]
  [ADD] -> Mux1/2
  CLEAR_ADD/1 -> Mux3/3

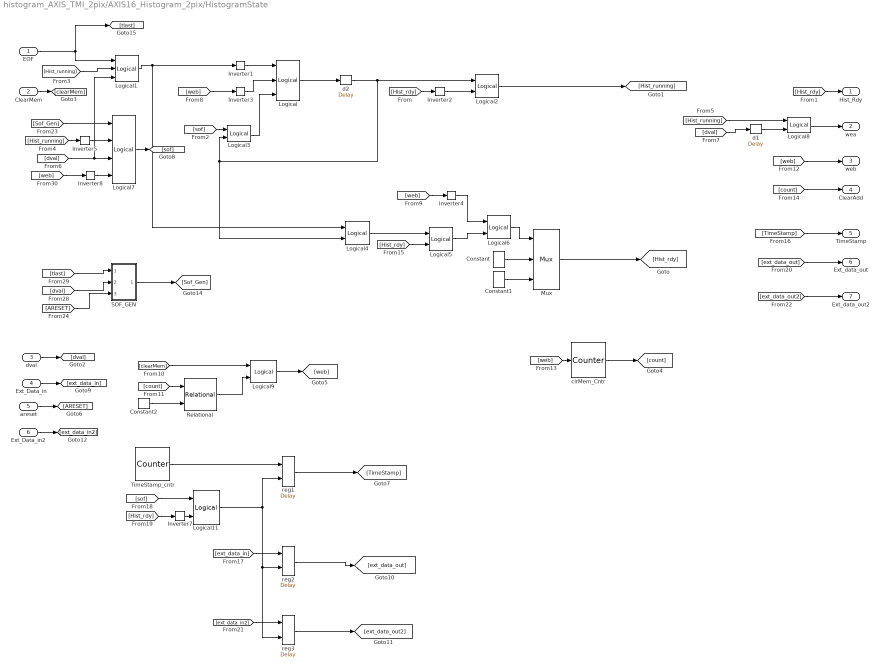
== system histogram_AXIS_TMI_2pix/AXIS16_Histogram_2pix/HistogramState ==
  EOF : Inport
  ClearMem : Inport  Port=2
  dval : Inport  Port=3
  Ext_Data_in : Inport  Port=4
  areset : Inport  Port=5
  Ext_Data_in2 : Inport  Port=6
  Constant : xbsIndex_r4/Constant  const=0  gui_display_data_type=Boolean  arith_type=Boolean  n_bits=16  bin_pt=14  preci_type=Single  exp_width=8  frac_width=24  explicit_period=off  period=1  equ=P=C  opselect=C  inp2=PCIN>>17  opr=+  inp1=P  carry=CIN  dbl_ovrd=off  block_type=constant
  Constant1 : xbsIndex_r4/Constant  const=1  gui_display_data_type=Boolean  arith_type=Boolean  n_bits=16  bin_pt=14  preci_type=Single  exp_width=8  frac_width=24  explicit_period=off  period=1  equ=P=C  opselect=C  inp2=PCIN>>17  opr=+  inp1=P  carry=CIN  dbl_ovrd=off  block_type=constant
  Constant2 : xbsIndex_r4/Constant  const=0  gui_display_data_type=Fixed-point  arith_type=Unsigned  n_bits=log2(Nb_bin)  bin_pt=0  preci_type=Single  exp_width=8  frac_width=24  explicit_period=off  period=1  equ=P=C  opselect=C  inp2=PCIN>>17  opr=+  inp1=P  carry=CIN  dbl_ovrd=off  block_type=constant
  Inverter{1..5,7..8} (7 alike) : xbsIndex_r4/Inverter  en=off  latency=0  dbl_ovrd=off  block_type=inv
      settings: xl_area=[0 0 0 0 0 0 0]
  Logical : xbsIndex_r4/Logical  logical_function=AND  inputs=3  en=off  latency=0  precision=Full  arith_type=Unsigned  n_bits=16  bin_pt=0  align_bp=on  dbl_ovrd=off  block_type=logical
      settings: xl_area=[1 0 0 1 0 0 0]
  Logical1 : xbsIndex_r4/Logical  logical_function=AND  inputs=3  en=off  latency=1  precision=Full  arith_type=Unsigned  n_bits=16  bin_pt=0  align_bp=on  dbl_ovrd=off  block_type=logical
      settings: xl_area=[1 1 0 1 0 0 0]
  Logical{2,4,6,8,11} (5 alike) : xbsIndex_r4/Logical  logical_function=AND  inputs=2  en=off  latency=0  precision=Full  arith_type=Unsigned  n_bits=16  bin_pt=0  align_bp=on  dbl_ovrd=off  block_type=logical
      settings: xl_area=[1 0 0 1 0 0 0]
  Logical3 : xbsIndex_r4/Logical  logical_function=OR  inputs=2  en=off  latency=0  precision=Full  arith_type=Unsigned  n_bits=16  bin_pt=0  align_bp=on  dbl_ovrd=off  block_type=logical
      settings: xl_area=[1 0 0 1 0 0 0]
  Logical5 : xbsIndex_r4/Logical  logical_function=OR  inputs=2  en=off  latency=0  precision=Full  arith_type=Unsigned  n_bits=16  bin_pt=0  align_bp=on  dbl_ovrd=off  block_type=logical
      settings: xl_area=[1 0 0 1 0 0 0]
  Logical7 : xbsIndex_r4/Logical  logical_function=AND  inputs=4  en=off  latency=0  precision=Full  arith_type=Unsigned  n_bits=16  bin_pt=0  align_bp=on  dbl_ovrd=off  block_type=logical
      settings: xl_area=[1 0 0 1 0 0 0]
  Logical9 : xbsIndex_r4/Logical  logical_function=OR  inputs=2  en=off  latency=0  precision=Full  arith_type=Unsigned  n_bits=16  bin_pt=0  align_bp=on  dbl_ovrd=off  block_type=logical
      settings: xl_area=[1 0 0 1 0 0 0]
  Mux : xbsIndex_r4/Mux  inputs=2  en=off  latency=1  precision=Full  arith_type=Unsigned  n_bits=16  bin_pt=14  quantization=Truncate  overflow=Wrap  dbl_ovrd=off  block_type=mux
      settings: xl_area=[1 1 0 1 0 0 0]
  Relational : xbsIndex_r4/Relational  mode=a!=b  op_type=Bool  en=off  latency=0  dbl_ovrd=off  block_type=relational
      settings: xl_area=[1 0 0 2 0 0 0]  block_version=10.1.3
  SOF_GEN : Subsystem
  TimeStamp_cntr : xbsIndex_r4/Counter  cnt_type=Free Running  cnt_to=Inf  operation=Up  start_count=0  cnt_by_val=1  arith_type=Unsigned  n_bits=32  bin_pt=0  load_pin=off  rst=off  en=off  explicit_period=on  period=1  use_behavioral_HDL=on  implementation=Fabric  use_rpm=off  dbl_ovrd=off  block_type=counter
  clrMem_Cntr : xbsIndex_r4/Counter  cnt_type=Count Limited  cnt_to=Nb_bin-1  operation=Up  start_count=0  cnt_by_val=1  arith_type=Unsigned  n_bits=log2(Nb_bin)  bin_pt=0  load_pin=off  rst=off  en=on  explicit_period=on  period=1  use_behavioral_HDL=off  implementation=Fabric  use_rpm=off  dbl_ovrd=off  block_type=counter
      settings: xl_area=[4 4 0 5 0 0 0]
  d1 : xbsIndex_r4/Delay  rst=off  infoeditControl=Selection of Reset will increase slice count due to use of real FFs and instead of SRLs  en=off  latency=1  reg_retiming=off  dbl_ovrd=off  block_type=delay
      settings: xl_area=[1 1 0 0 0 0 0]
  d2 : xbsIndex_r4/Delay  rst=off  infoeditControl=Selection of Reset will increase slice count due to use of real FFs and instead of SRLs  en=off  latency=1  reg_retiming=off  dbl_ovrd=off  block_type=delay
      settings: xl_area=[1 1 0 0 0 0 0]
  reg1 : xbsIndex_r4/Delay  rst=off  infoeditControl=Selection of Reset will increase slice count due to use of real FFs and instead of SRLs  en=on  latency=1  reg_retiming=off  dbl_ovrd=off  block_type=delay
      settings: xl_area=[1 1 0 0 0 0 0]
  reg2 : xbsIndex_r4/Delay  rst=off  infoeditControl=Selection of Reset will increase slice count due to use of real FFs and instead of SRLs  en=on  latency=1  reg_retiming=off  dbl_ovrd=off  block_type=delay
      settings: xl_area=[1 1 0 0 0 0 0]
  reg3 : xbsIndex_r4/Delay  rst=off  infoeditControl=Selection of Reset will increase slice count due to use of real FFs and instead of SRLs  en=on  latency=1  reg_retiming=off  dbl_ovrd=off  block_type=delay
      settings: xl_area=[1 1 0 0 0 0 0]
  Hist_Rdy : Outport
  wea : Outport  Port=2
  web : Outport  Port=3
  ClearAdd : Outport  Port=4
  TimeStamp : Outport  Port=5
  Ext_data_out : Outport  Port=6
  Ext_data_out2 : Outport  Port=7
  wires:
  Constant/1 -> Mux/2
  Constant1/1 -> Mux/3
  Mux/1 -> [Hist_rdy]
  Logical4/1 -> Logical5/1
  [Hist_rdy] -> Inverter2/1
  Inverter1/1 -> Logical/1
  Inverter3/1 -> Logical/2
  Logical3/1 -> Logical/3
  [Hist_rdy] -> Hist_Rdy/1
  [Hist_running] -> Logical1/2
  Logical1/1 -> Inverter1/1, Logical4/1
  Inverter5/1 -> Logical7/2
  [Hist_running] -> Inverter5/1
  Logical/1 -> d2/1
  d2/1 -> Logical3/2, Logical4/2, Logical2/1
  Inverter2/1 -> Logical2/2
  Logical2/1 -> [Hist_running]
  Logical8/1 -> wea/1
  [Hist_running] -> Logical8/1
  dval/1 -> [dval]
  [dval] -> Logical7/3, Logical1/3
  d1/1 -> Logical8/2
  [dval] -> d1/1
  ClearMem/1 -> [clearMem]
  [web] -> Inverter3/1
  [web] -> Inverter4/1
  [clearMem] -> Logical9/1
  Logical9/1 -> [web]
  Relational/1 -> Logical9/2
  Constant2/1 -> Relational/2
  clrMem_Cntr/1 -> [count]
  [count] -> Relational/1
  [web] -> web/1
  [web] -> clrMem_Cntr/1
  [count] -> ClearAdd/1
  [Hist_rdy] -> Logical5/2
  Logical6/1 -> Mux/1
  Inverter4/1 -> Logical6/1
  Logical5/1 -> Logical6/2
  areset/1 -> [ARESET]
  [TimeStamp] -> TimeStamp/1
  [sof] -> Logical11/1
  Logical11/1 -> reg1/2, reg2/2, reg3/2
  reg1/1 -> [TimeStamp]
  TimeStamp_cntr/1 -> reg1/1
  Logical7/1 -> [sof]
  [Hist_rdy] -> Inverter7/1
  Inverter7/1 -> Logical11/2
  [sof] -> Logical3/1
  Ext_Data_in/1 -> [ext_data_in]
  reg2/1 -> [ext_data_out]
  [ext_data_in] -> reg2/1
  [ext_data_out] -> Ext_data_out/1
  reg3/1 -> [ext_data_out2]
  [ext_data_in2] -> reg3/1
  Ext_Data_in2/1 -> [ext_data_in2]
  [ext_data_out2] -> Ext_data_out2/1
  [Sof_Gen] -> Logical7/1
  EOF/1 -> [tlast], Logical1/1
  [tlast] -> SOF_GEN/1(TLAST)
  [dval] -> SOF_GEN/2(DVAL)
  SOF_GEN/1(SOF) -> [Sof_Gen]
  Inverter8/1 -> Logical7/4
  [web] -> Inverter8/1
  [ARESET] -> SOF_GEN/3("ARESET ")

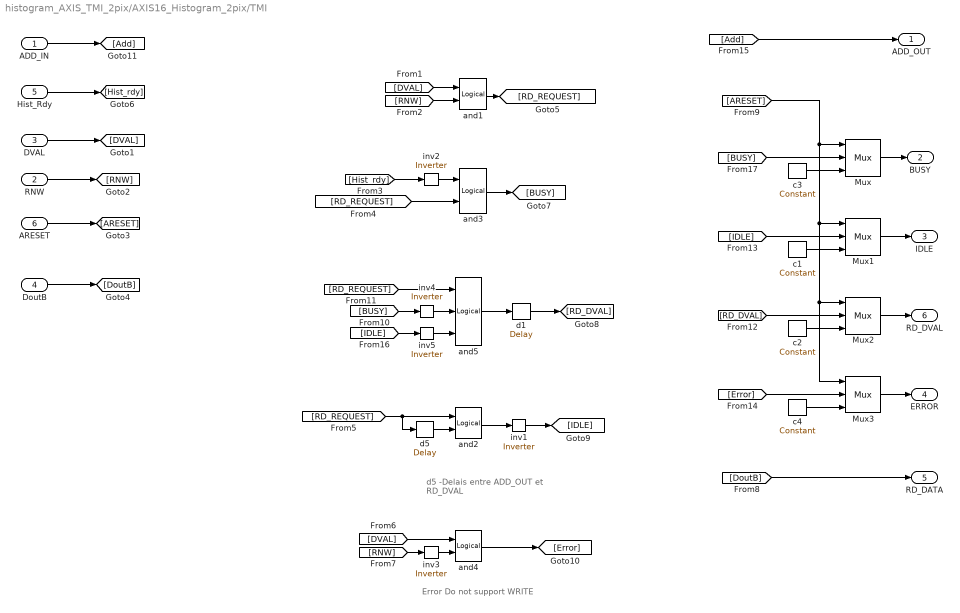
== system histogram_AXIS_TMI_2pix/AXIS16_Histogram_2pix/TMI ==
  note: d5 -Delais entre ADD_OUT
      |  et RD_DVAL
  note: Error Do not support WRITE
  ADD_IN : Inport
  RNW : Inport  Port=2
  DVAL : Inport  Port=3
  DoutB : Inport  Port=4
  Hist_Rdy : Inport  Port=5
  ARESET : Inport  Port=6
  Mux{,1..3} (4 alike) : xbsIndex_r4/Mux  inputs=2  en=off  latency=0  precision=Full  arith_type=Unsigned  n_bits=16  bin_pt=14  quantization=Truncate  overflow=Wrap  dbl_ovrd=off  block_type=mux
      settings: xl_area=[1 0 0 1 0 0 0]
  and1 : xbsIndex_r4/Logical  logical_function=AND  inputs=2  en=off  latency=0  precision=Full  arith_type=Unsigned  n_bits=16  bin_pt=0  align_bp=on  dbl_ovrd=off  block_type=logical
      settings: xl_area=[1 0 0 1 0 0 0]
  and2 : xbsIndex_r4/Logical  logical_function=OR  inputs=2  en=off  latency=0  precision=Full  arith_type=Unsigned  n_bits=16  bin_pt=0  align_bp=on  dbl_ovrd=off  block_type=logical
      settings: xl_area=[1 0 0 1 0 0 0]
  and3 : xbsIndex_r4/Logical  logical_function=AND  inputs=2  en=off  latency=0  precision=Full  arith_type=Unsigned  n_bits=16  bin_pt=0  align_bp=on  dbl_ovrd=off  block_type=logical
      settings: xl_area=[1 0 0 1 0 0 0]
  and4 : xbsIndex_r4/Logical  logical_function=AND  inputs=2  en=off  latency=0  precision=Full  arith_type=Unsigned  n_bits=16  bin_pt=0  align_bp=on  dbl_ovrd=off  block_type=logical
      settings: xl_area=[1 0 0 1 0 0 0]
  and5 : xbsIndex_r4/Logical  logical_function=AND  inputs=3  en=off  latency=0  precision=Full  arith_type=Unsigned  n_bits=16  bin_pt=0  align_bp=on  dbl_ovrd=off  block_type=logical
      settings: xl_area=[1 0 0 1 0 0 0]
  c1 : xbsIndex_r4/Constant  const=0  gui_display_data_type=Boolean  arith_type=Boolean  n_bits=MaxHistValue_bit  bin_pt=0  preci_type=Single  exp_width=8  frac_width=24  explicit_period=off  period=1  equ=P=C  opselect=C  inp2=PCIN>>17  opr=+  inp1=P  carry=CIN  dbl_ovrd=off  block_type=constant
  c2 : xbsIndex_r4/Constant  const=0  gui_display_data_type=Boolean  arith_type=Boolean  n_bits=MaxHistValue_bit  bin_pt=0  preci_type=Single  exp_width=8  frac_width=24  explicit_period=off  period=1  equ=P=C  opselect=C  inp2=PCIN>>17  opr=+  inp1=P  carry=CIN  dbl_ovrd=off  block_type=constant
  c3 : xbsIndex_r4/Constant  const=1  gui_display_data_type=Boolean  arith_type=Boolean  n_bits=MaxHistValue_bit  bin_pt=0  preci_type=Single  exp_width=8  frac_width=24  explicit_period=off  period=1  equ=P=C  opselect=C  inp2=PCIN>>17  opr=+  inp1=P  carry=CIN  dbl_ovrd=off  block_type=constant
  c4 : xbsIndex_r4/Constant  const=0  gui_display_data_type=Boolean  arith_type=Boolean  n_bits=MaxHistValue_bit  bin_pt=0  preci_type=Single  exp_width=8  frac_width=24  explicit_period=off  period=1  equ=P=C  opselect=C  inp2=PCIN>>17  opr=+  inp1=P  carry=CIN  dbl_ovrd=off  block_type=constant
  d1 : xbsIndex_r4/Delay  rst=off  infoeditControl=Selection of Reset will increase slice count due to use of real FFs and instead of SRLs  en=off  latency=1  reg_retiming=off  dbl_ovrd=off  block_type=delay
      settings: xl_area=[1 1 0 0 0 0 0]
  d5 : xbsIndex_r4/Delay  rst=off  infoeditControl=Selection of Reset will increase slice count due to use of real FFs and instead of SRLs  en=off  latency=1  reg_retiming=off  dbl_ovrd=off  block_type=delay
      settings: xl_area=[1 1 0 0 0 0 0]
  inv{1..5} (5 alike) : xbsIndex_r4/Inverter  en=off  latency=0  dbl_ovrd=off  block_type=inv
      settings: xl_area=[0 0 0 0 0 0 0]
  ADD_OUT : Outport
  BUSY : Outport  Port=2
  IDLE : Outport  Port=3
  ERROR : Outport  Port=4
  RD_DATA : Outport  Port=5
  RD_DVAL : Outport  Port=6
  wires:
  Hist_Rdy/1 -> [Hist_rdy]
  DVAL/1 -> [DVAL]
  RNW/1 -> [RNW]
  ARESET/1 -> [ARESET]
  DoutB/1 -> [DoutB]
  [DVAL] -> and1/1
  [RNW] -> and1/2
  d5/1 -> and2/2
  and2/1 -> inv1/1
  inv2/1 -> and3/1
  [Hist_rdy] -> inv2/1
  [RD_REQUEST] -> and3/2
  and1/1 -> [RD_REQUEST]
  [RD_REQUEST] -> and2/1, d5/1
  [DVAL] -> and4/1
  [RNW] -> inv3/1
  inv3/1 -> and4/2
  [DoutB] -> RD_DATA/1
  and3/1 -> [BUSY]
  [BUSY] -> inv4/1
  and5/1 -> d1/1
  d1/1 -> [RD_DVAL]
  inv1/1 -> [IDLE]
  and4/1 -> [Error]
  ADD_IN/1 -> [Add]
  [Add] -> ADD_OUT/1
  inv5/1 -> and5/3
  [IDLE] -> inv5/1
  Mux/1 -> BUSY/1
  [ARESET] -> Mux/1, Mux1/1, Mux2/1, Mux3/1
  [BUSY] -> Mux/2
  c3/1 -> Mux/3
  Mux1/1 -> IDLE/1
  [IDLE] -> Mux1/2
  c1/1 -> Mux1/3
  Mux2/1 -> RD_DVAL/1
  [RD_DVAL] -> Mux2/2
  c2/1 -> Mux2/3
  Mux3/1 -> ERROR/1
  [Error] -> Mux3/2
  c4/1 -> Mux3/3
  [RD_REQUEST] -> and5/1
  inv4/1 -> and5/2

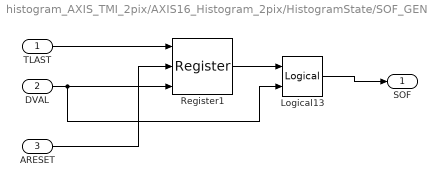
== system histogram_AXIS_TMI_2pix/AXIS16_Histogram_2pix/HistogramState/SOF_GEN ==
  TLAST : Inport
  DVAL : Inport  Port=2
  "ARESET " : Inport  Port=3
  Logical13 : xbsIndex_r4/Logical  logical_function=AND  inputs=2  en=off  latency=0  precision=Full  arith_type=Unsigned  n_bits=16  bin_pt=0  align_bp=on  dbl_ovrd=off  block_type=logical
      settings: xl_area=[1 0 0 1 0 0 0]
  Register1 : xbsIndex_r4/Register  init=1  rst=on  en=on  dbl_ovrd=off  block_type=register
  SOF : Outport
  wires:
  TLAST/1 -> Register1/1
  Register1/1 -> Logical13/1
  DVAL/1 -> Logical13/2, Register1/3
  Logical13/1 -> SOF/1
  "ARESET "/1 -> Register1/2
